simulink model "closed_loop"  (R2016b)
settings: Solver=VariableStepAuto  StartTime=0.0  StopTime=10.0  RelTol=1e-3
values from neighbouring files (symbols this model uses):
  A = [0      1              0           0 ... (first row only)    [ImportStateSpace.m]    (also in multi_plot_tune_observer.m = sys.A; multi_plot_tune_observer2.m = sys.A; responseObserver.m = sys.A)
  B = [     0 ... (first row only)    [ImportStateSpace.m]    (also in multi_plot_tune_observer.m = sys.B; multi_plot_tune_observer2.m = sys.B; responseObserver.m = sys.B)
  C = [1 0 0 0 ... (first row only)    [ImportStateSpace.m]    (also in multi_plot_tune_observer.m = sys.C; multi_plot_tune_observer2.m = sys.C; responseObserver.m = sys.C)
  D = zeros(size(C,1), size(B,2))    [ImportStateSpace.m]    (also in multi_plot_tune_observer.m = sys.D; multi_plot_tune_observer2.m = sys.D; responseObserver.m = sys.D)
  K = place(sys.A, sys.B, eigs)    [LCSproject.m]    (also in myLQR.m = lqr(sys.A, sys.B, Q, R))
  kr = -1/(C*inv(A-B*K)*B)    [LCSproject.m]
  L = place(A',C',P)'    [LCSproject.m]    (also in drawCartPend.m = 2; multi_plot_tune_observer.m = place(A',C',Poles)'; multi_plot_tune_observer2.m = place(A',C',Poles)')
libraries: simulink x1
settings Model: Creator=Olivier  LastModifiedBy=Olivier

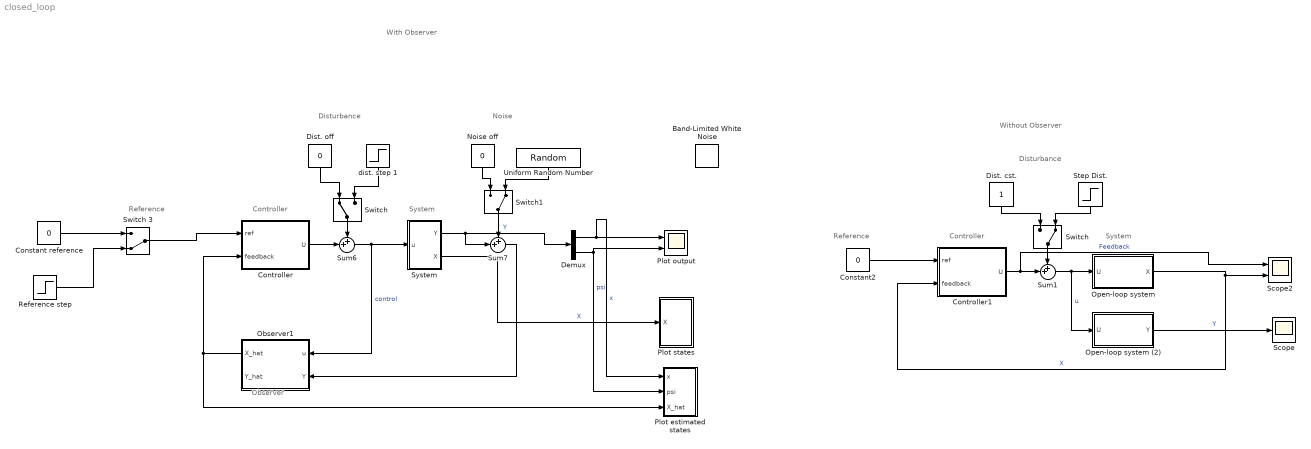
== system closed_loop ==
  note: With Observer
  note: System
  note: Observer
  note: Controller
  note: Reference
  note: Disturbance
  note: Noise
  note: System
  note: Controller
  note: Reference
  note: Disturbance
  note: Without Observer
  " Switch" : ManualSwitch
  Band-Limited White Noise : simulink/Sources/Band-Limited White Noise  Cov=[0.00001, 0.00001]  Ts=0.1  seed=[23341]
  Constant reference : Constant  Value=0
  Constant2 : Constant  Value=0
  Controller : Subsystem
  Controller1 : Subsystem
  Demux : Demux  Outputs=2
  Dist. cst. : Constant
  Dist. off : Constant  Value=0
  Noise off : Constant  Value=0
  Observer1 : Subsystem
  Open-loop system : Subsystem
  Open-loop system (2) : Subsystem
  Plot estimated states : Subsystem
  Plot output : Scope  NumInputPorts=2
  Plot states : Subsystem
  Reference step : Step  Time=0.2  After=0.2  SampleTime=0
  Scope : Scope
  Scope2 : Scope  NumInputPorts=2
  Step Dist. : Step  After=0.2  SampleTime=0
  Sum1 : Sum  Inputs=++|
  Sum6 : Sum  Inputs=++|
  Sum7 : Sum  Inputs=++|
  Switch : ManualSwitch  CurrentSetting=0
  Switch 3 : ManualSwitch  CurrentSetting=0
  Switch1 : ManualSwitch  CurrentSetting=0
  System : Subsystem
  Uniform Random Number : UniformRandomNumber  Minimum=-0.005  Maximum=0.005  SampleTime=0.1
  dist. step 1 : Step  Time=0.2  SampleTime=0
  wires:
  Controller/1(U) -> Sum6/2
  Observer1/1(X_hat) -> Plot estimated states/3(X_hat), Controller/2(feedback)
  Sum6/1 -> Observer1/1(u), System/1(u)  "control"
  Open-loop system/1(X) -> Scope2/2, Controller1/2(feedback)  "X"
  Controller1/1(U) -> Scope2/1, Sum1/2  "Feedback"
  Sum1/1 -> Open-loop system (2)/1(U), Open-loop system/1(U)  "u"
  Dist. cst./1 -> Switch/1
  Constant reference/1 -> Switch 3/1
  Open-loop system (2)/1(Y) -> Scope/1  "Y"
  Constant2/1 -> Controller1/1(ref)
  dist. step 1/1 -> " Switch"/2
  " Switch"/1 -> Sum6/1
  Dist. off/1 -> " Switch"/1
  Switch1/1 -> Sum7/1
  Noise off/1 -> Switch1/1
  Demux/2 -> Plot estimated states/2(psi), Plot output/2  "psi"
  Demux/1 -> Plot estimated states/1(x), Plot output/1  "x"
  System/1(Y) -> Demux/1, Sum7/2  "Y"
  System/2(X) -> Plot states/1(X)  "X"
  Switch/1 -> Sum1/1
  Step Dist./1 -> Switch/2
  Switch 3/1 -> Controller/1(ref)
  Reference step/1 -> Switch 3/2
  Sum7/1 -> Observer1/2(Y)
  Uniform Random Number/1 -> Switch1/2

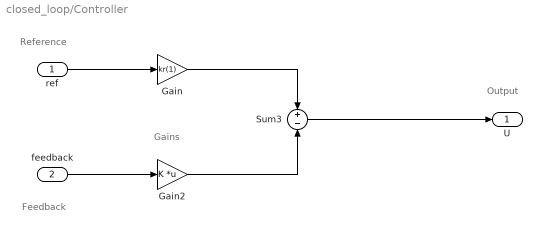
== system closed_loop/Controller ==
  note: Output
  note: Gains
  note: Feedback
  note: Reference
  ref : Inport
  feedback : Inport  Port=2
  Gain : Gain  Gain=kr(1)
  Gain2 : Gain  Gain=K  Multiplication=Matrix(K*u)
  Sum3 : Sum  Inputs=+|-
  U : Outport
  wires:
  Sum3/1 -> U/1
  Gain2/1 -> Sum3/2
  feedback/1 -> Gain2/1
  ref/1 -> Gain/1
  Gain/1 -> Sum3/1

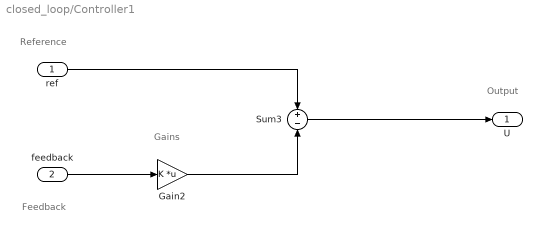
== system closed_loop/Controller1 ==
  note: Output
  note: Gains
  note: Feedback
  note: Reference
  ref : Inport
  feedback : Inport  Port=2
  Gain2 : Gain  Gain=K  Multiplication=Matrix(K*u)
  Sum3 : Sum  Inputs=+|-
  U : Outport
  wires:
  Sum3/1 -> U/1
  Gain2/1 -> Sum3/2
  feedback/1 -> Gain2/1
  ref/1 -> Sum3/1

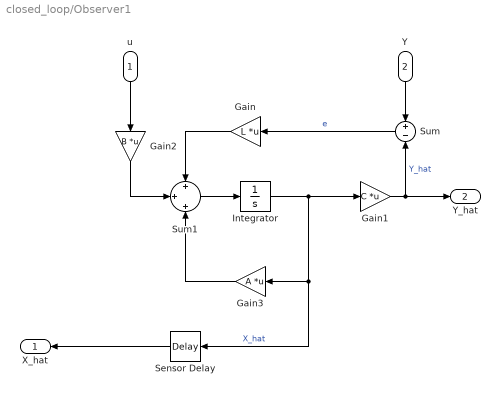
== system closed_loop/Observer1 ==
  u : Inport
  Y : Inport  Port=2
  Gain : Gain  Gain=L  Multiplication=Matrix(K*u)
  Gain1 : Gain  Gain=C  Multiplication=Matrix(K*u)
  Gain2 : Gain  Gain=B  Multiplication=Matrix(K*u)
  Gain3 : Gain  Gain=A  Multiplication=Matrix(K*u)
  Integrator : Integrator
  Sensor Delay : TransportDelay  DelayTime=0.01
  Sum : Sum  Inputs=+|-
  Sum1 : Sum  Inputs=+|+|+
  X_hat : Outport
  Y_hat : Outport  Port=2
  wires:
  Sum/1 -> Gain/1  "e"
  Y/1 -> Sum/1
  Sum1/1 -> Integrator/1
  Integrator/1 -> Sensor Delay/1, Gain3/1, Gain1/1  "X_hat"
  Gain1/1 -> Y_hat/1, Sum/2  "Y_hat"
  Gain/1 -> Sum1/1
  u/1 -> Gain2/1
  Gain2/1 -> Sum1/2
  Gain3/1 -> Sum1/3
  Sensor Delay/1 -> X_hat/1

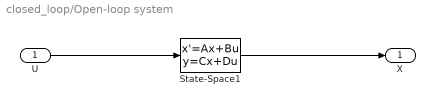
== system closed_loop/Open-loop system ==
  U : Inport
  State-Space1 : StateSpace  A=A  B=B  C=eye(4)  D=[0;0;0;0]  X0=0
  X : Outport
  wires:
  U/1 -> State-Space1/1
  State-Space1/1 -> X/1

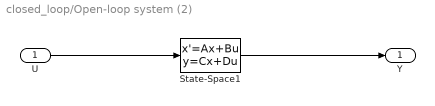
== system closed_loop/Open-loop system (2) ==
  U : Inport
  State-Space1 : StateSpace  A=A  B=B  C=C  D=D  X0=0
  Y : Outport
  wires:
  U/1 -> State-Space1/1
  State-Space1/1 -> Y/1

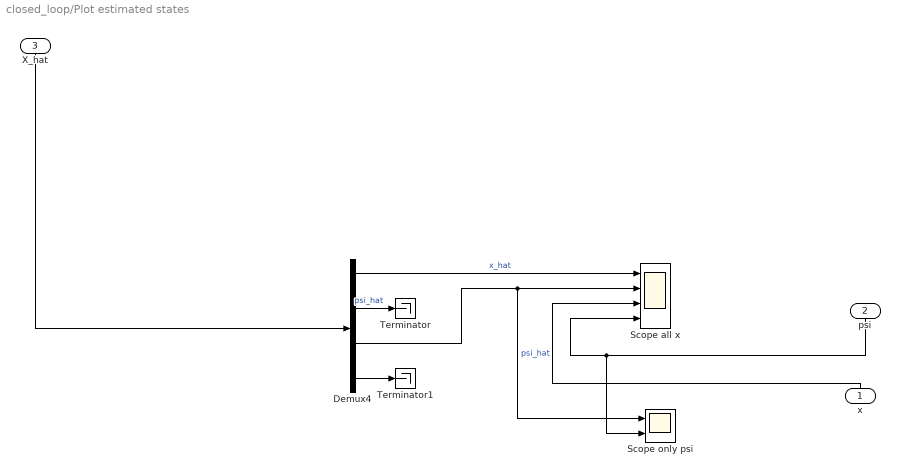
== system closed_loop/Plot estimated states ==
  x : Inport
  psi : Inport  Port=2
  X_hat : Inport  Port=3
  Demux4 : Demux
  Scope all x : Scope  NumInputPorts=4
  Scope only psi : Scope  NumInputPorts=2
  Terminator : Terminator
  Terminator1 : Terminator
  wires:
  Demux4/2 -> Terminator/1  "psi_hat"
  Demux4/3 -> Scope only psi/1, Scope all x/2  "psi_hat"
  Demux4/1 -> Scope all x/1  "x_hat"
  psi/1 -> Scope only psi/2, Scope all x/4
  x/1 -> Scope all x/3
  X_hat/1 -> Demux4/1
  Demux4/4 -> Terminator1/1

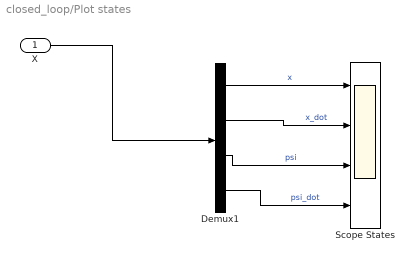
== system closed_loop/Plot states ==
  X : Inport
  Demux1 : Demux
  Scope States : Scope  NumInputPorts=4
  wires:
  Demux1/4 -> Scope States/4  "psi_dot"
  Demux1/3 -> Scope States/3  "psi"
  Demux1/2 -> Scope States/2  "x_dot"
  Demux1/1 -> Scope States/1  "x"
  X/1 -> Demux1/1

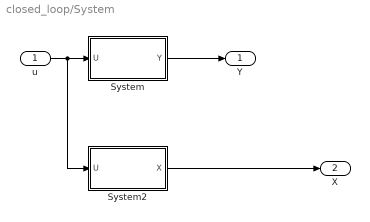
== system closed_loop/System ==
  u : Inport
  System : Subsystem
  System2 : Subsystem
  Y : Outport
  X : Outport  Port=2
  wires:
  System2/1(X) -> X/1
  System/1(Y) -> Y/1
  u/1 -> System2/1(U), System/1(U)

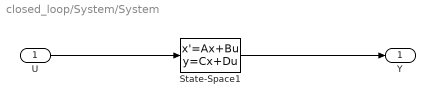
== system closed_loop/System/System ==
  U : Inport
  State-Space1 : StateSpace  A=A  B=B  C=C  D=D  X0=0
  Y : Outport
  wires:
  U/1 -> State-Space1/1
  State-Space1/1 -> Y/1

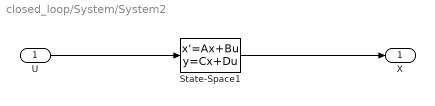
== system closed_loop/System/System2 ==
  U : Inport
  State-Space1 : StateSpace  A=A  B=B  C=eye(4)  D=[0;0;0;0]  X0=0
  X : Outport
  wires:
  U/1 -> State-Space1/1
  State-Space1/1 -> X/1
